simulink model "uni_model_discrete1"  (R2017b)
settings: Solver=FixedStepDiscrete  StartTime=0.0  StopTime=20  FixedStep=dt  RelTol=1e-3
values from neighbouring files (symbols this model uses):
  dt = 0.1    [extendedKalmanFilter.m]    (also in matlab.mat; runV3.m; rungen.m; runpathfollower.m)
libraries: simulink x3
settings Model: Creator=nisha  LastModifiedBy=nisha

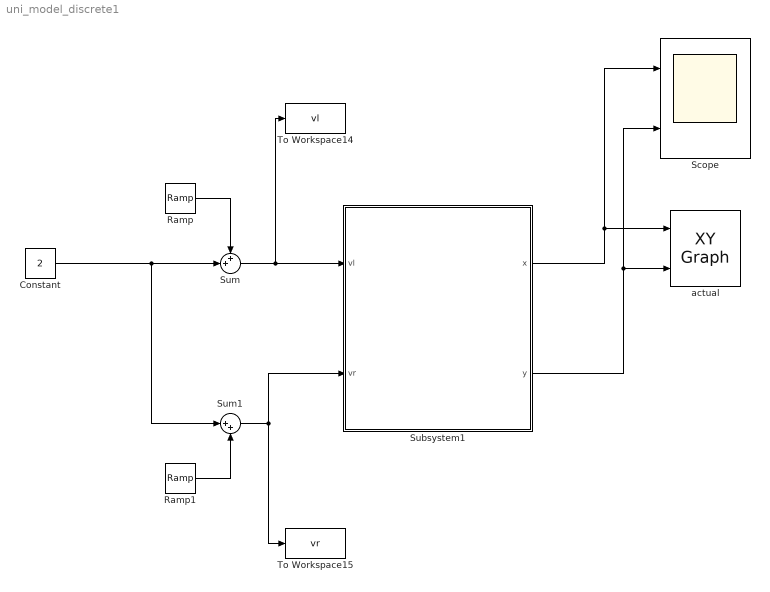
== system uni_model_discrete1 ==
  Constant : Constant  Value=2
  Ramp : simulink/Sources/Ramp  slope=0.1  start=2  X0=0
  Ramp1 : simulink/Sources/Ramp  slope=0.1  start=3  X0=0
  Scope : Scope  NumInputPorts=2
  Subsystem1 : Subsystem
  Sum : Sum  Inputs=++|
  Sum1 : Sum  Inputs=|++
  To Workspace14 : ToWorkspace  VariableName=vl  SampleTime=-1
  To Workspace15 : ToWorkspace  VariableName=vr  SampleTime=-1
  actual : simulink/Sinks/XY Graph  xmin=-5  xmax=10  ymin=-10  ymax=5  st=-1
  wires:
  Ramp1/1 -> Sum1/2
  Sum1/1 -> Subsystem1/2(vr), To Workspace15/1
  Constant/1 -> Sum1/1, Sum/2
  Ramp/1 -> Sum/1
  Sum/1 -> Subsystem1/1(vl), To Workspace14/1
  Subsystem1/1(x) -> Scope/1, actual/1
  Subsystem1/2(y) -> Scope/2, actual/2

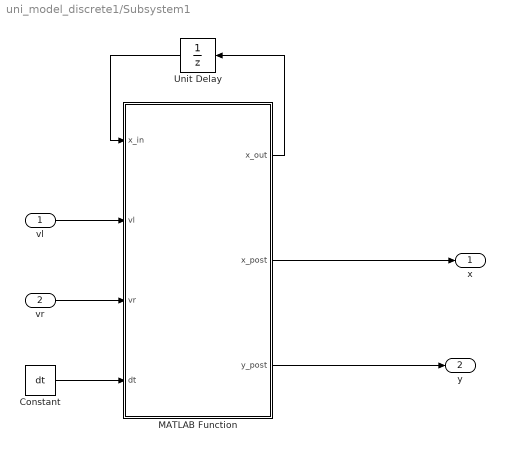
== system uni_model_discrete1/Subsystem1 ==
  vl : Inport
  vr : Inport  Port=2
  Constant : Constant  Value=dt
  MATLAB Function : MATLAB Function  TreatAsAtomicUnit=on
  Unit Delay : UnitDelay  InitialCondition=[0;0;0;0;0;0;0;0]  SampleTime=-1
  x : Outport
  y : Outport  Port=2
  wires:
  vl/1 -> MATLAB Function/2(vl)
  MATLAB Function/1(x_out) -> Unit Delay/1
  Unit Delay/1 -> MATLAB Function/1(x_in)
  vr/1 -> MATLAB Function/3(vr)
  MATLAB Function/2(x_post) -> x/1
  MATLAB Function/3(y_post) -> y/1
  Constant/1 -> MATLAB Function/4(dt)

== matlab function uni_model_discrete1/Subsystem1/MATLAB Function ==
  data: x_in input; x_out output; vl input; vr input; x_post output; y_post output; dt input
function [x_out,x_post,y_post]         = fcn(x_in,vl, vr,dt)

d=0.15;
x=x_in(1); y=x_in(2); dx=x_in(3);dy=x_in(4);ddx=x_in(5);ddy=x_in(6); phi=x_in(7); dphi=x_in(8);
th=phi+0.5*dphi*dt;
x_out = ...
[x + dx*dt + ddx*dt^2/2
 y + dy*dt + ddy*dt^2/2
 (vl+vr)/2*cos(th)+ddx*dt
 (vl+vr)/2*sin(th)+ddy*dt
 ddx
 ddy
 phi + dphi*dt
 (vr-vl)/d];

x_post=x_out(1); y_post=x_out(2);
end
